simulink model "controle_discreto_pv"  (R2022a)
settings: Solver=FixedStepDiscrete  StartTime=0.0  StopTime=30  FixedStep=0.01  RelTol=1e-3
undefined symbols (not defined in the file or in its folder): Hden, Hnum
settings Model: Creator=phcs  LastModifiedBy=phcs

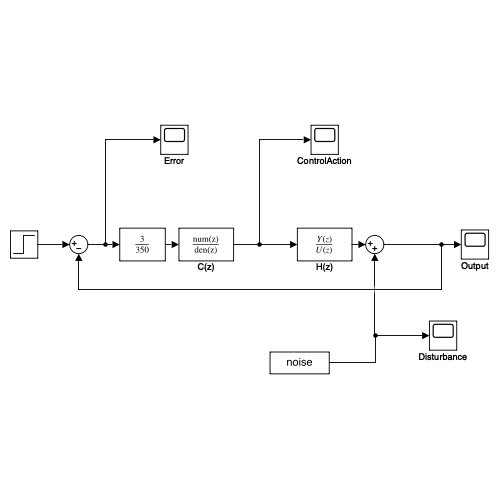
[thumbnail: Simulink's stored preview of the top-level diagram]
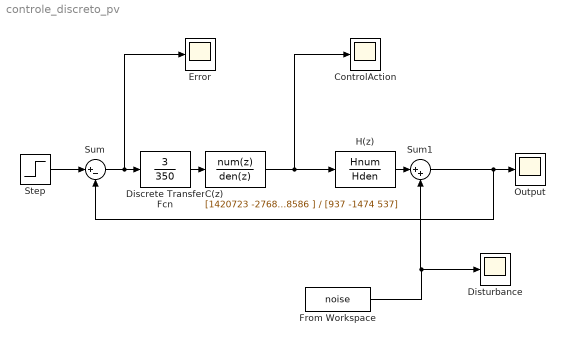
== system controle_discreto_pv ==
  C(z) : DiscreteTransferFcn  Numerator=[1420723 -2768909 1348586 ]  Denominator=[937 -1474 537]
  ControlAction : Scope
  Discrete Transfer Fcn : DiscreteTransferFcn  Numerator=[3]  Denominator=[350]
  Disturbance : Scope
  Error : Scope
  From Workspace : FromWorkspace  VariableName=noise
  H(z) : DiscreteTransferFcn  Numerator=Hnum  Denominator=Hden
  Output : Scope
  Step : Step  After=0  SampleTime=0
  Sum : Sum  Inputs=|+-
  Sum1 : Sum  Inputs=|++
  wires:
  Sum1/1 -> Sum/2, Output/1
  Sum/1 -> Discrete Transfer Fcn/1, Error/1
  Step/1 -> Sum/1
  C(z)/1 -> H(z)/1, ControlAction/1
  Discrete Transfer Fcn/1 -> C(z)/1
  H(z)/1 -> Sum1/1
  From Workspace/1 -> Sum1/2, Disturbance/1
